simulink model "PWM_Rectifier_3phase"  (Simulink 7.4)
settings: Solver=ode45  StartTime=0.0  StopTime=0.1  MaxStep=2e-6  RelTol=1e-3
InitFcn:
  | clear;
  | clc;
  | f=50;
  | Vp=110;
  | fs=10e3;
  | k=1.2;
libraries: powerlib x21, simulink x1
settings Model: Creator=Syed Abdul Rahman  LastModifiedBy=Syed Abdul Rahman

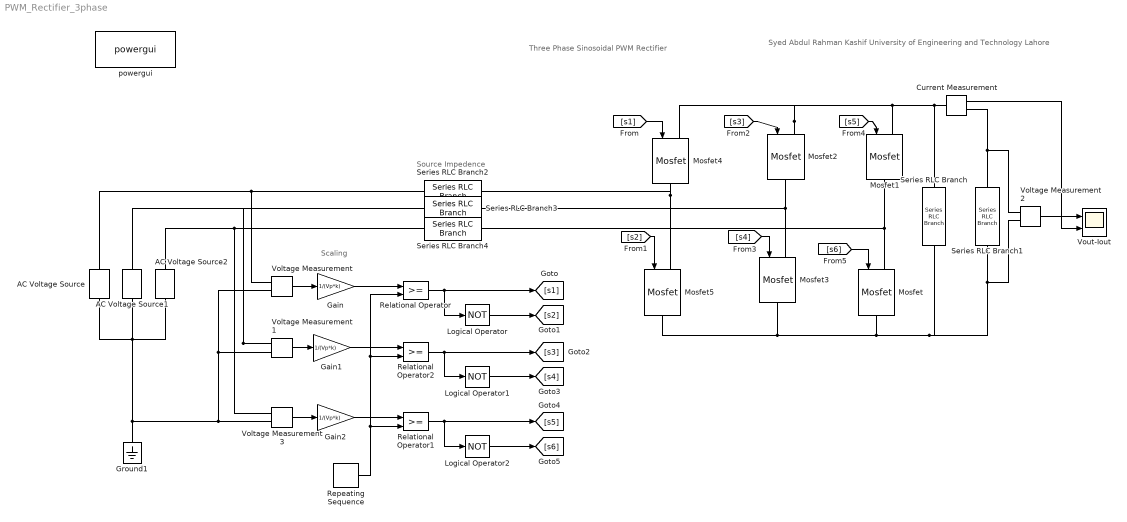
== system PWM_Rectifier_3phase ==
  note: Three Phase Sinosoidal PWM Rectifier
  note: Syed Abdul Rahman Kashif
      | University of Engineering and Technology
      | Lahore
  note: Source Impedence
  note: Scaling
  AC Voltage Source : powerlib/Electrical Sources/AC Voltage Source  DialogController=POWERSYS.PowerSysDialog  SystemSampleTime=-1  Amplitude=Vp  Phase=0  Frequency=f  SampleTime=0  Measurements=None
  AC Voltage Source1 : powerlib/Electrical Sources/AC Voltage Source  DialogController=POWERSYS.PowerSysDialog  SystemSampleTime=-1  Amplitude=Vp  Phase=240  Frequency=f  SampleTime=0  Measurements=None
  AC Voltage Source2 : powerlib/Electrical Sources/AC Voltage Source  DialogController=POWERSYS.PowerSysDialog  SystemSampleTime=-1  Amplitude=Vp  Phase=120  Frequency=f  SampleTime=0  Measurements=None
  Current Measurement : powerlib/Measurements/Current Measurement  DialogController=POWERSYS.PowerSysDialog  SystemSampleTime=-1  PhasorSimulation=off  OutputType=Complex  PSBequivalent=0
  Gain : Gain  Gain=1/(Vp*k)  ParameterDataType=fixdt(1, 16)  ParameterScaling=2^0  OutDataType=fixdt(1, 16)  OutScaling=2^0
  Gain1 : Gain  Gain=1/(Vp*k)  ParameterDataType=fixdt(1, 16)  ParameterScaling=2^0  OutDataType=fixdt(1, 16)  OutScaling=2^0
  Gain2 : Gain  Gain=1/(Vp*k)  ParameterDataType=fixdt(1, 16)  ParameterScaling=2^0  OutDataType=fixdt(1, 16)  OutScaling=2^0
  Ground1 : powerlib/Elements/Ground  DialogController=POWERSYS.PowerSysDialog  PhysicalDomain=powersysdomain  SubClassName=unknown  LeftPortType=p1  RightPortType=p1  LConnTagsString=a
  Logical Operator : Logic  Operator=NOT  AllPortsSameDT=off  OutDataTypeMode=boolean  LogicDataType=fixdt(0, 8)  OutDataTypeStr=boolean
  Logical Operator1 : Logic  Operator=NOT  AllPortsSameDT=off  OutDataTypeMode=boolean  LogicDataType=fixdt(0, 8)  OutDataTypeStr=boolean
  Logical Operator2 : Logic  Operator=NOT  AllPortsSameDT=off  OutDataTypeMode=boolean  LogicDataType=fixdt(0, 8)  OutDataTypeStr=boolean
  Mosfet{,1..5} (6 alike) : powerlib/Power Electronics/Mosfet  DialogController=POWERSYS.PowerSysDialog  SystemSampleTime=-1  Ron=0.1  Lon=0  Rd=0.01  Vfd=0  IC=0  Rs=1e5  Cs=inf  Measurements=off
  Relational Operator : RelationalOperator  LogicOutDataTypeMode=boolean  LogicDataType=fixdt(0, 8)  OutDataTypeStr=boolean
  Relational Operator1 : RelationalOperator  LogicOutDataTypeMode=boolean  LogicDataType=fixdt(0, 8)  OutDataTypeStr=boolean
  Relational Operator2 : RelationalOperator  LogicOutDataTypeMode=boolean  LogicDataType=fixdt(0, 8)  OutDataTypeStr=boolean
  Repeating Sequence : simulink/Sources/Repeating Sequence  SystemSampleTime=-1  rep_seq_t=[0 0.25/fs 0.5/fs 0.75/fs 1/fs]  rep_seq_y=[0 -1 0 1 0]
  Series RLC Branch : powerlib/Elements/Series RLC Branch  DialogController=POWERSYS.PowerSysDialog  PhysicalDomain=powersysdomain  SubClassName=unknown  LeftPortType=p1  RightPortType=p1  LConnTagsString=__new0  RConnTagsString=__new0  BranchType=C  Resistance=5  Inductance=1e-3  SetiL0=off  InitialCurrent=0  Capacitance=470e-6  Setx0=off  InitialVoltage=0  Measurements=None
  Series RLC Branch1 : powerlib/Elements/Series RLC Branch  DialogController=POWERSYS.PowerSysDialog  PhysicalDomain=powersysdomain  SubClassName=unknown  LeftPortType=p1  RightPortType=p1  LConnTagsString=__new0  RConnTagsString=__new0  BranchType=RL  Resistance=5  Inductance=1e-3  SetiL0=off  InitialCurrent=0  Capacitance=200e-6  Setx0=off  InitialVoltage=0  Measurements=None
  Series RLC Branch2 : powerlib/Elements/Series RLC Branch  DialogController=POWERSYS.PowerSysDialog  PhysicalDomain=powersysdomain  SubClassName=unknown  LeftPortType=p1  RightPortType=p1  LConnTagsString=__new0  RConnTagsString=__new0  BranchType=RL  Resistance=0.5  Inductance=1e-3  SetiL0=off  InitialCurrent=0  Capacitance=200e-6  Setx0=off  InitialVoltage=0  Measurements=None
  Series RLC Branch3 : powerlib/Elements/Series RLC Branch  DialogController=POWERSYS.PowerSysDialog  PhysicalDomain=powersysdomain  SubClassName=unknown  LeftPortType=p1  RightPortType=p1  LConnTagsString=__new0  RConnTagsString=__new0  BranchType=RL  Resistance=0.5  Inductance=1e-3  SetiL0=off  InitialCurrent=0  Capacitance=200e-6  Setx0=off  InitialVoltage=0  Measurements=None
  Series RLC Branch4 : powerlib/Elements/Series RLC Branch  DialogController=POWERSYS.PowerSysDialog  PhysicalDomain=powersysdomain  SubClassName=unknown  LeftPortType=p1  RightPortType=p1  LConnTagsString=__new0  RConnTagsString=__new0  BranchType=RL  Resistance=0.5  Inductance=1e-3  SetiL0=off  InitialCurrent=0  Capacitance=200e-6  Setx0=off  InitialVoltage=0  Measurements=None
  Voltage Measurement{,1..3} (4 alike) : powerlib/Measurements/Voltage Measurement  DialogController=POWERSYS.PowerSysDialog  SystemSampleTime=-1  PhasorSimulation=off  OutputType=Complex  PSBequivalent=0
  Vout-Iout : Scope  NumInputPorts=2
      settings: YMin=0~0  YMax=210~40  SaveName=Vout  MaxDataPoints=5000000  SampleInput=on  SampleTime=2e-6
  powergui : powerlib/powergui  Priority=1  SystemSampleTime=-1  SimulationMode=Discrete  SampleTime=2e-6  frequency=60  SPID=off  DisableSnubberDevices=off  DisableRonSwitches=off  DisableVfSwitches=off  SwTol=0  Interpol=off  frequencyindice=50  echomessages=off  HookPort=off  DisplayEquations=off  FunctionMessages=off  EnableUseOfTLC=off  x0status=blocks  RestoreLinks=warning  Frange=[0:2:500]  Ylog=off  Xlog=on  ShowGrid=off  save=off  variable=ZData  ZoomFFT=on  StartTime=0.0  cycles=1  DisplayStyle=1  fundamental=60  FreqAxis=off  MaxFrequency=1000  frequencyindicesteady=1  RmsSteady=1  display=off  Ts=0  methode=off
  wires:
  [s1] -> Mosfet4/1
  [s2] -> Mosfet5/1
  [s3] -> Mosfet2/1
  [s4] -> Mosfet3/1
  [s5] -> Mosfet1/1
  [s6] -> Mosfet/1
  Voltage Measurement/1 -> Gain/1
  Voltage Measurement3/1 -> Gain2/1
  Voltage Measurement1/1 -> Gain1/1
  Voltage Measurement2/1 -> Vout-Iout/1
  Repeating Sequence/1 -> Relational Operator1/2, Relational Operator2/2, Relational Operator/2
  Relational Operator/1 -> [s1], Logical Operator/1
  Logical Operator/1 -> [s2]
  Relational Operator2/1 -> [s3], Logical Operator1/1
  Logical Operator1/1 -> [s4]
  Relational Operator1/1 -> [s5], Logical Operator2/1
  Logical Operator2/1 -> [s6]
  Gain/1 -> Relational Operator/1
  Gain1/1 -> Relational Operator2/1
  Gain2/1 -> Relational Operator1/1
  Current Measurement/1 -> Vout-Iout/2
  connections:
  Series RLC Branch/LConn1 -- Mosfet1/LConn1 -- Mosfet2/LConn1 -- Mosfet4/LConn1 -- Current Measurement/LConn1
  Mosfet4/RConn1 -- Mosfet5/LConn1 -- Series RLC Branch2/LConn1
  Mosfet/LConn1 -- Mosfet1/RConn1 -- Series RLC Branch4/LConn1
  Series RLC Branch1/RConn1 -- Mosfet3/RConn1 -- Mosfet5/RConn1 -- Mosfet/RConn1 -- Series RLC Branch/RConn1 -- Voltage Measurement2/LConn2
  Mosfet2/RConn1 -- Mosfet3/LConn1 -- Series RLC Branch3/LConn1
  AC Voltage Source/LConn1 -- AC Voltage Source1/LConn1 -- AC Voltage Source2/LConn1 -- Voltage Measurement1/LConn2 -- Voltage Measurement/LConn2 -- Voltage Measurement3/LConn2 -- Ground1/LConn1
  Voltage Measurement/LConn1 -- AC Voltage Source/RConn1 -- Series RLC Branch2/RConn1
  Voltage Measurement1/LConn1 -- AC Voltage Source1/RConn1 -- Series RLC Branch3/RConn1
  Voltage Measurement3/LConn1 -- AC Voltage Source2/RConn1 -- Series RLC Branch4/RConn1
  Current Measurement/RConn1 -- Series RLC Branch1/LConn1 -- Voltage Measurement2/LConn1
